simulink model "pulse_generator"  (R2016b)
settings: Solver=FixedStepAuto  StartTime=0.0  StopTime=100.0  RelTol=1e-3
settings Model: Creator=hbourbou  LastModifiedBy=hbourbou

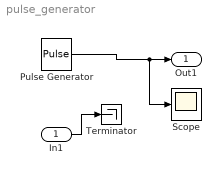
== system pulse_generator ==
  In1 : Inport
  Pulse Generator : DiscretePulseGenerator  PulseType=Time based  Period=10  PulseWidth=5  PhaseDelay=4
  Scope : Scope
  Terminator : Terminator
  Out1 : Outport
  wires:
  Pulse Generator/1 -> Scope/1, Out1/1
  In1/1 -> Terminator/1
